simulink model "Simulation_model_full"  (R2021a)
settings: Solver=ode23t  StartTime=0.0  StopTime=6  FixedStep=T  RelTol=1e-3
values from neighbouring files (symbols this model uses):
  C_dc = Cb*c_dc_pu    [parameters.m]
  C_f = Cb*c_f_pu    [parameters.m]
  f_SM = fb    (= 50)    [parameters.m]
  fb = 50    [parameters.m]
  ff_SM = 0.01322    [parameters.m]
  Ib = 2/3*Sb/Vb    [parameters.m]
  Ib_dc = Sb/Vb_dc    [parameters.m]
  ic_SM = 0.8    [parameters.m]
  K_ad = 1.5    [parameters.m]
  K_ffv = 0    [parameters.m]
  K_ic = K_pc/T_1    [parameters.m]
  K_idc = K_pdc/T_idc    (= 250)    [parameters.m]
  K_iPLL = a^2*T_fPLL    (= 0.09)    [parameters.m]
  K_iv = K_pv/T_iv    (= 92.0050761421)    [parameters.m]
  K_iv_SM = K_pv_SM/T_iv_SM    (= 70)    [parameters.m]
  K_omega = 20    [parameters.m]
  K_omega_SM = 40    [parameters.m]
  K_pc = l_f_pu/(4*pi*fb*T_sum)    (= 1.27323954474)    [parameters.m]
  K_pdc = 25    [parameters.m]
  K_pPLL = 1/(a*2*pi*T_fPLL)    (= 5.30516476973)    [parameters.m]
  K_pv = 0.29    [parameters.m]
  K_pv_SM = 35    [parameters.m]
  K_vco = 2*pi    (= 6.28318530718)    [parameters.m]
  Kd = 40    [parameters.m]
  Kq = 0.1    [parameters.m]
  Kq_SM = 0.1    [parameters.m]
  L_f = Lb*l_f_pu    [parameters.m]
  l_f_pu = 0.08    [parameters.m]
  lfd_SM = 0.531    [parameters.m]
  llkd = 2.655    [parameters.m]
  llkq1 = 0.2408    [parameters.m]
  lls_SM = 0.08    [parameters.m]
  lmd_SM = 2.81    [parameters.m]
  lmq_SM = 1.64    [parameters.m]
  omega_ad = 50    [parameters.m]
  omega_b = 2*pi*fb    (= 314.159265359)    [parameters.m]
  omega_d = 5    [parameters.m]
  omega_qf = 200    [parameters.m]
  omega_qf_SM = 200    [parameters.m]
  omega_vf = 200    [parameters.m]
  p_h = 0.1    [parameters.m]
  pp_SM = 2    [parameters.m]
  R_lf = Rb*r_lf_pu    [parameters.m]
  rfd_SM = 0.004319    [parameters.m]
  rkd = 0.2343    [parameters.m]
  rkq1 = 0.03365    [parameters.m]
  rs_SM = 0.01524    [parameters.m]
  S_SM = Sb    (= 1000000)    [parameters.m]
  Sb = 1e6    (= 1000000)    [parameters.m]
  T = 1e-4    (= 0.0001)    [parameters.m]
  T_fPLL = 10e-3    (= 0.01)    [parameters.m]
  T_gt_SM = 0.5    [parameters.m]
  Ta = 4    [parameters.m]
  V_dc_bat = 1200    [parameters.m]
  v_dc_ref = 1    [parameters.m]
  V_SM = V    (= 690)    [parameters.m]
  Vb = V*sqrt(2)/sqrt(3)    [parameters.m]
  Vb_dc = Vb*2    [parameters.m]
undefined symbols (not defined in the file or in its folder): D1, Delta
libraries: simulink_extras x36, spsDiodeLib x24, spsThreePhaseVIMeasurementLib x16, spsThreePhaseSeriesRLCBranchLib x14, spsPower3phInstantaneousLib x8, spsVoltageMeasurementLib x5, spsControlledCurrentSourceLib x4, spsUniversalBridgeLib x4, spsParallelRLCBranchLib x2, spsSeriesRLCBranchLib x2, spsSynchronousMachinepuFundamentalLib x2, spsThreePhaseParallelRLCLoadLib x2
(part 1 of 3)
settings Model: Creator=HLunn  LastModifiedBy=HLunn

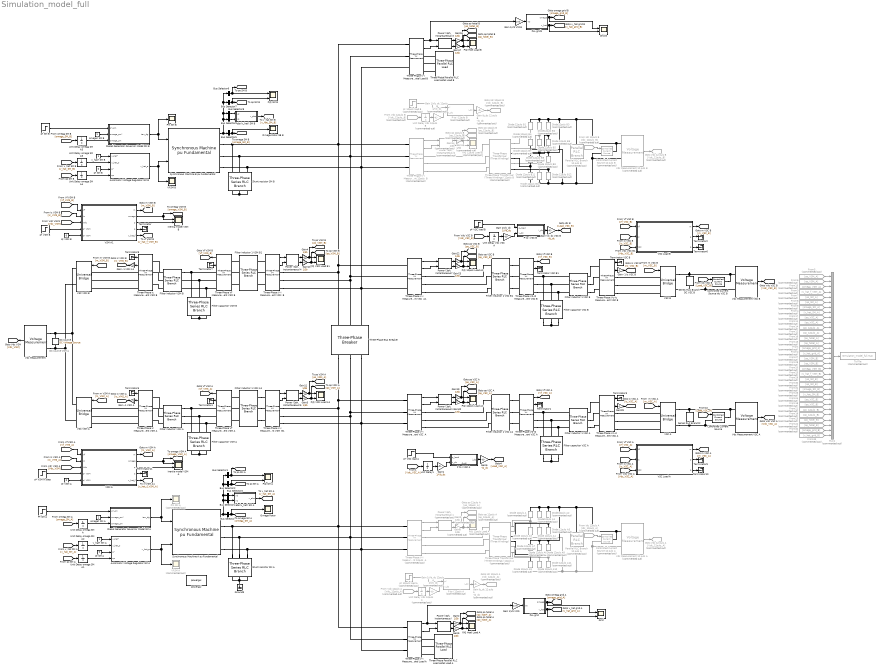
== system Simulation_model_full ==
  note: DC source
      | VSM A
  Automatic Voltage Regulator SM A : Subsystem
  Automatic Voltage Regulator SM B : Subsystem
  Bus Selector : BusSelector  OutputSignals="Mechanical.Rotor speed  wm (pu)"  OutputAsBus=on
  Bus Selector1 : BusSelector  OutputSignals="Output active power   Peo (pu)"  OutputAsBus=on
  Bus Selector2 : BusSelector  OutputSignals="Output reactive power  Qeo (pu)"  OutputAsBus=on
  Bus Selector3 : BusSelector  OutputSignals="dq0 components.Stator voltage  vd (pu)"  OutputAsBus=on
  Bus Selector4 : BusSelector  OutputSignals="dq0 components.Stator voltage  vq (pu)"  OutputAsBus=on
  Bus Selector5 : BusSelector  OutputSignals="Mechanical.Rotor speed  wm (pu)"  OutputAsBus=on
  Bus Selector6 : BusSelector  OutputSignals="Output active power   Peo (pu)"  OutputAsBus=on
  Bus Selector7 : BusSelector  OutputSignals="Output reactive power  Qeo (pu)"  OutputAsBus=on
  Bus Selector8 : BusSelector  OutputSignals="dq0 components.Stator voltage  vd (pu)"  OutputAsBus=on
  Bus Selector9 : BusSelector  OutputSignals="dq0 components.Stator voltage  vq (pu)"  OutputAsBus=on
  Controlled Current Source : spsControlledCurrentSourceLib/Controlled Current Source  Initialize=on  Source_Type=DC  Amplitude=0  Phase=0  Frequency=0  Measurements=None
  Controlled Current Source 12 puls A : spsControlledCurrentSourceLib/Controlled Current Source  Commented=on  Initialize=on  Source_Type=DC  Amplitude=0  Phase=0  Frequency=0  Measurements=None
  Controlled Current Source 12 puls B : spsControlledCurrentSourceLib/Controlled Current Source  Commented=on  Initialize=on  Source_Type=DC  Amplitude=0  Phase=0  Frequency=0  Measurements=None
  Controlled Current Source Idc VSC B : spsControlledCurrentSourceLib/Controlled Current Source  Initialize=on  Source_Type=DC  Amplitude=0  Phase=0  Frequency=0  Measurements=None
  DC source : spsDCVoltageSourceLib/DC Voltage Source  Amplitude=V_dc_bat  Measurements=None
  Diesel Generator Governor Model SM A : Subsystem
  Diesel Generator Governor Model SM B : Subsystem
  Diode 12puls A{,3..11} (10 alike) : spsDiodeLib/Diode  Commented=on  Ron=0.001  Lon=0  Vf=0.8  IC=0  UseSnubber=0  Rs=500  Cs=250e-9  Measurements=off
  Diode 12puls B{1,4..12} (10 alike) : spsDiodeLib/Diode  Commented=on  Ron=0.001  Lon=0  Vf=0.8  IC=0  UseSnubber=0  Rs=500  Cs=250e-9  Measurements=off
  Diode12puls A1 : spsDiodeLib/Diode  Commented=on  Ron=0.001  Lon=0  Vf=0.8  IC=0  UseSnubber=0  Rs=500  Cs=250e-9  Measurements=off
  Diode12puls A2 : spsDiodeLib/Diode  Commented=on  Ron=0.001  Lon=0  Vf=0.8  IC=0  UseSnubber=0  Rs=500  Cs=250e-9  Measurements=off
  Diode12puls B2 : spsDiodeLib/Diode  Commented=on  Ron=0.001  Lon=0  Vf=0.8  IC=0  UseSnubber=0  Rs=500  Cs=250e-9  Measurements=off
  Diode12puls B3 : spsDiodeLib/Diode  Commented=on  Ron=0.001  Lon=0  Vf=0.8  IC=0  UseSnubber=0  Rs=500  Cs=250e-9  Measurements=off
  Filter capacitor VSC A : spsThreePhaseSeriesRLCBranchLib/Three-Phase Series RLC Branch  LConnTagsString=A|B|C  RConnTagsString=A|B|C  BranchType=C  Resistance=R_lf*0  Inductance=L_f  Capacitance=C_f  Measurements=None
  Filter capacitor VSC B : spsThreePhaseSeriesRLCBranchLib/Three-Phase Series RLC Branch  LConnTagsString=A|B|C  RConnTagsString=A|B|C  BranchType=C  Resistance=R_lf*0  Inductance=L_f  Capacitance=C_f  Measurements=None
  Filter capacitor VSM A : spsThreePhaseSeriesRLCBranchLib/Three-Phase Series RLC Branch  LConnTagsString=A|B|C  RConnTagsString=A|B|C  BranchType=C  Resistance=R_lf*0  Inductance=L_f  Capacitance=C_f  Measurements=None
  Filter capacitor VSM B : spsThreePhaseSeriesRLCBranchLib/Three-Phase Series RLC Branch  LConnTagsString=A|B|C  RConnTagsString=A|B|C  BranchType=C  Resistance=R_lf*0  Inductance=L_f  Capacitance=C_f  Measurements=None
  Filter inductor VSM A : spsThreePhaseSeriesRLCBranchLib/Three-Phase Series RLC Branch  LConnTagsString=A|B|C  RConnTagsString=A|B|C  BranchType=RL  Resistance=R_lf  Inductance=L_f  Capacitance=1e-6  Measurements=None
  Filter inductor VSM B : spsThreePhaseSeriesRLCBranchLib/Three-Phase Series RLC Branch  LConnTagsString=A|B|C  RConnTagsString=A|B|C  BranchType=RL  Resistance=R_lf  Inductance=L_f  Capacitance=1e-6  Measurements=None
  Filter inductor 1 VSC A : spsThreePhaseSeriesRLCBranchLib/Three-Phase Series RLC Branch  LConnTagsString=A|B|C  RConnTagsString=A|B|C  BranchType=RL  Resistance=R_lf  Inductance=L_f  Capacitance=1e-6  Measurements=None
  Filter inductor 1 VSC A1 : spsThreePhaseSeriesRLCBranchLib/Three-Phase Series RLC Branch  LConnTagsString=A|B|C  RConnTagsString=A|B|C  BranchType=RL  Resistance=R_lf  Inductance=L_f  Capacitance=1e-6  Measurements=None
  Filter inductor 1 VSC B : spsThreePhaseSeriesRLCBranchLib/Three-Phase Series RLC Branch  LConnTagsString=A|B|C  RConnTagsString=A|B|C  BranchType=RL  Resistance=R_lf  Inductance=L_f  Capacitance=1e-6  Measurements=None
  Filter inductor 1 VSC B1 : spsThreePhaseSeriesRLCBranchLib/Three-Phase Series RLC Branch  LConnTagsString=A|B|C  RConnTagsString=A|B|C  BranchType=RL  Resistance=R_lf  Inductance=L_f  Capacitance=1e-6  Measurements=None
  Filter inductor 1 VSM A1 : spsThreePhaseSeriesRLCBranchLib/Three-Phase Series RLC Branch  LConnTagsString=A|B|C  RConnTagsString=A|B|C  BranchType=RL  Resistance=R_lf  Inductance=L_f  Capacitance=1e-6  Measurements=None
  Filter inductor 1 VSM B1 : spsThreePhaseSeriesRLCBranchLib/Three-Phase Series RLC Branch  LConnTagsString=A|B|C  RConnTagsString=A|B|C  BranchType=RL  Resistance=R_lf  Inductance=L_f  Capacitance=1e-6  Measurements=None
  From : From  Commented=on  GotoTag=omega_grid_A
  From Idc 12puls A : From  Commented=on  GotoTag=Idc_12puls_A
  From Idc 12puls B : From  Commented=on  GotoTag=Idc_12puls_B
  From Vdc 12puls A : From  Commented=on  GotoTag=Vdc_12puls_A
  From Vdc 12puls B : From  Commented=on  GotoTag=Vdc_12puls_B
  From11 : From  Commented=on  GotoTag=qo_VSC_A
  From12 : From  Commented=on  GotoTag=qo_12puls_A
  From13 : From  Commented=on  GotoTag=omega_VSM_A
  From14 : From  Commented=on  GotoTag=po_12puls_A
  From15 : From  Commented=on  GotoTag=qo_hotel_A
  From16 : From  Commented=on  GotoTag=po_hotel_A
  From17 : From  Commented=on  GotoTag=po_VSC_A
  From18 : From  Commented=on  GotoTag=qo_VSC_B
  From19 : From  Commented=on  GotoTag=qo_12puls_B
  From2 : From  Commented=on  GotoTag=v_hat_grid_A
  From20 : From  Commented=on  GotoTag=omega_VSM_B
  From21 : From  Commented=on  GotoTag=po_12puls_B
  From22 : From  Commented=on  GotoTag=qo_hotel_B
  From23 : From  Commented=on  GotoTag=po_hotel_B
  From24 : From  Commented=on  GotoTag=po_VSC_B
  From25 : From  Commented=on  GotoTag=v_hat_f_VSM_B
  From26 : From  Commented=on  GotoTag=v_hat_SM_B
  From27 : From  Commented=on  GotoTag=po_VSM_B
  From28 : From  Commented=on  GotoTag=qo_VSM_B
  From29 : From  Commented=on  GotoTag=po_SM_B
  From3 : From  Commented=on  GotoTag=v_hat_f_VSM_A
  From30 : From  Commented=on  GotoTag=qo_SM_B
  From31 : From  Commented=on  GotoTag=omega_SM_B
  From32 : From  Commented=on  GotoTag=omega_grid_B
  From33 : From  Commented=on  GotoTag=v_hat_grid_B
  From4 : From  Commented=on  GotoTag=v_hat_SM_A
  From5 : From  Commented=on  GotoTag=po_VSM_A
  From6 : From  Commented=on  GotoTag=qo_VSM_A
  From7 : From  Commented=on  GotoTag=po_SM_A
  From8 : From  Commented=on  GotoTag=qo_SM_A
  From9 : From  Commented=on  GotoTag=omega_SM_A
  Gain -1 Ic VSC B : Gain  Gain=-1
  Gain -1 VSM A : Gain  Gain=-1
  Gain -1 VSM A1 : Gain  Gain=-1
  Gain 1/Vb VMS : Gain  Gain=1/Vb
  Gain 1/Vb VMS1 : Gain  Gain=1/Vb
  Gain 1/Vb_dc : Gain  Gain=1/Vb_dc
  Gain 1/Vb_dc 12puls A : Gain  Commented=on  Gain=1/Vb_dc
  Gain 1/Vb_dc 12puls B : Gain  Commented=on  Gain=1/Vb_dc
  Gain Ib_dc 12 puls A : Gain  Commented=on  Gain=-Ib_dc
  Gain Ib_dc 12 puls B : Gain  Commented=on  Gain=-Ib_dc
  Gain Vb_dc VSC B : Gain  Gain=-Ib_dc
  Gain1 : Gain  Gain=1/Vb_dc
  Gain{2..5,10..11,16..17,19..20,22..23} (12 alike) : Gain  Gain=1/Sb
  Gain{8..9,13..14} (4 alike) : Gain  Commented=on  Gain=1/Sb
  Gain29 : Gain  Gain=-1
  Gain6 : Gain  Gain=-Ib_dc
  Goto Idc 12puls A : Goto  Commented=on  GotoTag=Idc_12puls_A
  Goto Idc 12puls B : Goto  Commented=on  GotoTag=Idc_12puls_B
  Goto Vdc 12 puls A : Goto  Commented=on  GotoTag=Vdc_12puls_A
  Goto Vdc 12 puls B : Goto  Commented=on  GotoTag=Vdc_12puls_B
  Goto po 12puls A : Goto  Commented=on  GotoTag=po_12puls_A
  Goto po 12puls B : Goto  Commented=on  GotoTag=po_12puls_B
  Goto qo 12puls A : Goto  Commented=on  GotoTag=qo_12puls_A
  Goto qo 12puls B : Goto  Commented=on  GotoTag=qo_12puls_B
  Grid : Scope  NumInputPorts=2
  Grid B : Scope  NumInputPorts=2
  Ground3 : spsGroundLib/Ground  LConnTagsString=a
  Inertia model VSM A : Scope  NumInputPorts=2
  Inertia model VSM B : Scope  NumInputPorts=2
  Mux1 : Mux  Commented=on  Inputs=32
  Omega Rotor : Scope
  Omega Rotor SB B : Scope
  P to I VSC A : Subsystem
      settings: PortSchema="{\"entries\":[{\"content\":{\"sides\":[{\"content\":{\"connectorIds\":[\"In1\",\"In2\"]},\"type\":\"ConnectorPlacement.EquallySpacedRectSide\",\"uuid\":\"1b3d670f-a973-44e5-93e0-282aed06b720\"},{\"content\":{\"connectorIds\":[\"Out1\"],\"side\":\"RIGHT\"},\"type\":\"ConnectorPlacement.EquallySpacedRectSide\",\"uuid\":\"c6dbaf48-01df-4046-a8d4-fcaf539dec06\"},{\"content\":{\"connectorIds\":[],\"side\":\"TOP\"},\"type\":\"ConnectorPlacement.EquallySpacedRectSide\",\"uuid\":\"017adae8-c967-4395-bb40-0db2b451d960\"},{\"content\":{\"connectorIds\":[\"Out2\"],\"side\":\"BOTTOM\"},\"type\":\"ConnectorPlacement.EquallySpacedRectSide\",\"uuid\":\"114f5234-785a-4230-ad61-b1c2a38e27d5\"}]},\"type\":\"ConnectorPlacement.EquallySpacedConnector\",\"uuid\":\"a79c07b6-0122-49d2-8cca-a205e7e92776\"}],\"packageUris\":[\"http://schema.mathworks.com/mf0/Connector/R2020b\"],\"version\":\"1.0\"}"
  P to I VSC B : Subsystem
  P to I 12puls A : Subsystem  Commented=on
  P to I 12puls B : Subsystem  Commented=on
  "P* SM A " : Step  Time=2  Before=0.05  After=0.2  SampleTime=0
  P/Q 12puls Load A : Scope  Commented=on  NumInputPorts=2
  P/Q 12puls Load A1 : Scope  NumInputPorts=2
  P/Q 12puls Load A2 : Scope  NumInputPorts=2
  P/Q 12puls Load B : Scope  Commented=on  NumInputPorts=2
  P/Q Hoel Load A : Scope  NumInputPorts=2
  P/Q Hoel Load B : Scope  NumInputPorts=2
  P/Q SM A : Scope  NumInputPorts=2
  P/Q SM B : Scope  NumInputPorts=2
  P/Q VSM Load A1 : Scope  NumInputPorts=2
  P/Q VSM Load B1 : Scope  NumInputPorts=2
  PLL grid : Subsystem
  PLL grid1 : Subsystem
  Parallel RLC Branch 12 puls A : spsParallelRLCBranchLib/Parallel RLC Branch  Commented=on  LConnTagsString=a  RConnTagsString=__new0  BranchType=C  Resistance=1e3  Inductance=1e-3  SetiL0=off  InitialCurrent=0  Capacitance=C_dc  Setx0=on  InitialVoltage=Vb_dc  Measurements=None
  Parallel RLC Branch 12 puls B : spsParallelRLCBranchLib/Parallel RLC Branch  Commented=on  LConnTagsString=a  RConnTagsString=__new0  BranchType=C  Resistance=1e3  Inductance=1e-3  SetiL0=off  InitialCurrent=0  Capacitance=C_dc  Setx0=on  InitialVoltage=Vb_dc  Measurements=None
  Pm SM A : Scope  Commented=on
  Pm SM B : Scope
  Power (3ph, Instantaneous){,3..7} (6 alike) : spsPower3phInstantaneousLib/Power (3ph, Instantaneous)
  "Power (3ph, Instantaneous)1" : spsPower3phInstantaneousLib/Power (3ph, Instantaneous)  Commented=on
  "Power (3ph, Instantaneous)2" : spsPower3phInstantaneousLib/Power (3ph, Instantaneous)  Commented=on
  Series RLC Branch DC VSC B : spsSeriesRLCBranchLib/Series RLC Branch  LConnTagsString=__new0  RConnTagsString=__new0  BranchType=C  Resistance=0  Inductance=0  SetiL0=off  InitialCurrent=0  Capacitance=C_dc  Setx0=on  InitialVoltage=Vb_dc  Measurements=None
  Series RLC Branch2 : spsSeriesRLCBranchLib/Series RLC Branch  LConnTagsString=__new0  RConnTagsString=__new0  BranchType=C  Resistance=0  Inductance=0  SetiL0=off  InitialCurrent=0  Capacitance=C_dc  Setx0=on  InitialVoltage=Vb_dc  Measurements=None
  Shunt resistor SM A : spsThreePhaseSeriesRLCBranchLib/Three-Phase Series RLC Branch  LConnTagsString=A|B|C  RConnTagsString=A|B|C  BranchType=R  Resistance=1e6  Inductance=L_f  Capacitance=C_f  Measurements=None
  Shunt resistor SM B : spsThreePhaseSeriesRLCBranchLib/Three-Phase Series RLC Branch  LConnTagsString=A|B|C  RConnTagsString=A|B|C  BranchType=R  Resistance=1e6  Inductance=L_f  Capacitance=C_f  Measurements=None
  Synchronous Machine A pu Fundamental : spsSynchronousMachinepuFundamentalLib/Synchronous Machine pu Fundamental  PresetModel=No  MechanicalLoad=Mechanical power Pm  ShowDetailedParameters=on  RotorType=Salient-pole  Units=per unit fundamental parameters  MeasurementBus=off  NominalParameters=[S_SM V_SM f_SM]  Stator=[rs_SM lls_SM lmd_SM lmq_SM]  Field=[rfd_SM lfd_SM]  Dampers2=[0.0652, 0.5134, 0.0287, 0.2553, 7.765e-3, 0.9167 ]  Dampers1=[rkd llkd rkq1 llkq1]  Mechanical=[ic_SM ff_SM pp_SM]  PolePairs=20  InitialConditions="[ 0  0  0  0  0  0  0  0  1 ]"  SetSaturation=off  Saturation=[0.6404,0.7127,0.8441,0.9214,0.9956,1.082,1.19,1.316,1.457;0.7,0.7698,0.8872,0.9466,0.9969,1.046,1.1,1.151,1.201]  LoadFlowParameters=[1,0,0,0,0]  TsPowergui=0  TsBlock=-1  IterativeModel=Trapezoidal non iterative  IterativeDiscreteModel=Trapezoidal non iterative  BusType=PV  Pref=0  Qref=0  Qmin=-inf  Qmax=inf  PLF=0  QLF=0
      settings: SourceProductBaseCode=PS
  Synchronous Machine B pu Fundamental : spsSynchronousMachinepuFundamentalLib/Synchronous Machine pu Fundamental  PresetModel=No  MechanicalLoad=Mechanical power Pm  ShowDetailedParameters=on  RotorType=Salient-pole  Units=per unit fundamental parameters  MeasurementBus=off  NominalParameters=[S_SM V_SM f_SM]  Stator=[rs_SM lls_SM lmd_SM lmq_SM]  Field=[rfd_SM lfd_SM]  Dampers2=[0.0652, 0.5134, 0.0287, 0.2553, 7.765e-3, 0.9167 ]  Dampers1=[rkd llkd rkq1 llkq1]  Mechanical=[ic_SM ff_SM pp_SM]  PolePairs=20  InitialConditions="[ 0  0  0  0  0  0  0  0  1 ]"  SetSaturation=off  Saturation=[0.6404,0.7127,0.8441,0.9214,0.9956,1.082,1.19,1.316,1.457;0.7,0.7698,0.8872,0.9466,0.9969,1.046,1.1,1.151,1.201]  LoadFlowParameters=[1,0,0,0,0]  TsPowergui=0  TsBlock=-1  IterativeModel=Trapezoidal non iterative  IterativeDiscreteModel=Trapezoidal non iterative  BusType=PV  Pref=0  Qref=0  Qmin=-inf  Qmax=inf  PLF=0  QLF=0
      settings: SourceProductBaseCode=PS
  Terminator{,1..11} (12 alike) : Terminator
  Terminator VSC B : Terminator
  Terminator VSC B1 : Terminator
  Three-Phase Ic Measurement VSM A : spsThreePhaseVIMeasurementLib/Three-Phase V-I Measurement  VoltageMeasurement=phase-to-ground  SetLabelV=off  LabelV=V_cv  Vpu=off  VpuLL=off  CurrentMeasurement=yes  SetLabelI=off  LabelI=I_cv  Ipu=off  Pbase=Sb  Vbase=V  OutputType=Complex  PhasorSimulation=off  PSBequivalent=0
  Three-Phase Ic Measurement VSM B : spsThreePhaseVIMeasurementLib/Three-Phase V-I Measurement  VoltageMeasurement=phase-to-ground  SetLabelV=off  LabelV=V_cv  Vpu=off  VpuLL=off  CurrentMeasurement=yes  SetLabelI=off  LabelI=I_cv  Ipu=off  Pbase=Sb  Vbase=V  OutputType=Complex  PhasorSimulation=off  PSBequivalent=0
  Three-Phase Parallel RLC Load Hotel Load A : spsThreePhaseParallelRLCLoadLib/Three-Phase Parallel RLC Load  LConnTagsString=A|B|C  Configuration=Y (floating)  NominalVoltage=690  Vabc=[1e3 1e3 1e3]  Vabcp=[1e3 1e3 1e3]  NominalFrequency=fb  UnbalancedPower=off  ActivePower=Sb*p_h  InductivePower=0  CapacitivePower=0  Pabc=[10e3 9e3 11e3]  QLabc=[100 90 110]  QCabc=[100 90 110]  Pabcp=[10e3 9e3 11e3]  QLabcp=[100 90 110]  QCabcp=[100 90 110]  Measurements=None  LoadType=constant Z
  Three-Phase Parallel RLC Load Hotel Load B : spsThreePhaseParallelRLCLoadLib/Three-Phase Parallel RLC Load  LConnTagsString=A|B|C  Configuration=Y (floating)  NominalVoltage=690  Vabc=[1e3 1e3 1e3]  Vabcp=[1e3 1e3 1e3]  NominalFrequency=fb  UnbalancedPower=off  ActivePower=Sb*p_h  InductivePower=0  CapacitivePower=0  Pabc=[10e3 9e3 11e3]  QLabc=[100 90 110]  QCabc=[100 90 110]  Pabcp=[10e3 9e3 11e3]  QLabcp=[100 90 110]  QCabcp=[100 90 110]  Measurements=None  LoadType=constant Z
  Three-Phase Transformer (Three Windings) 12puls A : spsThreePhaseTransformerThreeWindingsLib/Three-Phase Transformer (Three Windings)  Commented=on  Winding1Connection=Y  Winding2Connection=Y  Winding3Connection=Delta (D1)  CoreType=Three single-phase transformers  SetSaturation=off  Hysteresis=off  DataFile='hysteresis'  SetInitialFlux=off  Measurements=None  UNITS=pu  NominalPower=[Sb , fb]  Winding1=[690 0.005 0.04]  Winding2=[690 0.005 0.03]  Winding3=[690 0.005 0.03]  Rm=100  Lm=100  L0=0.5  Saturation=[0 0;2.2531e-06 1278.3;0.00093879 1619.1]  InitialFluxes=[0.8 -0.8 0.7]  BreakLoop=off  DiscreteSolver=Trapezoidal iterative  DataType=off  TransfoNumber=1
      settings: SourceProductBaseCode=PS
  Three-Phase Transformer (Three Windings) 12puls B : spsThreePhaseTransformerThreeWindingsLib/Three-Phase Transformer (Three Windings)  Commented=on  Winding1Connection=Y  Winding2Connection=Y  Winding3Connection=Delta (D1)  CoreType=Three single-phase transformers  SetSaturation=off  Hysteresis=off  DataFile='hysteresis'  SetInitialFlux=off  Measurements=None  UNITS=pu  NominalPower=[Sb , fb]  Winding1=[690 0.005 0.04]  Winding2=[690 0.005 0.03]  Winding3=[690 0.005 0.03]  Rm=100  Lm=100  L0=0.5  Saturation=[0 0;2.2531e-06 1278.3;0.00093879 1619.1]  InitialFluxes=[0.8 -0.8 0.7]  BreakLoop=off  DiscreteSolver=Trapezoidal iterative  DataType=off  TransfoNumber=1
      settings: SourceProductBaseCode=PS
  Three-Phase V-I Measurement 12puls  A : spsThreePhaseVIMeasurementLib/Three-Phase V-I Measurement  Commented=on  VoltageMeasurement=phase-to-ground  SetLabelV=off  LabelV=Vabc  Vpu=off  VpuLL=off  CurrentMeasurement=yes  SetLabelI=off  LabelI=Iabc  Ipu=off  Pbase=100e6  Vbase=500e3  OutputType=Complex  PhasorSimulation=off  PSBequivalent=0
  Three-Phase V-I Measurement 12puls  B : spsThreePhaseVIMeasurementLib/Three-Phase V-I Measurement  Commented=on  VoltageMeasurement=phase-to-ground  SetLabelV=off  LabelV=Vabc  Vpu=off  VpuLL=off  CurrentMeasurement=yes  SetLabelI=off  LabelI=Iabc  Ipu=off  Pbase=100e6  Vbase=500e3  OutputType=Complex  PhasorSimulation=off  PSBequivalent=0
  Three-Phase V-I Measurement Hotel Load A : spsThreePhaseVIMeasurementLib/Three-Phase V-I Measurement  VoltageMeasurement=phase-to-ground  SetLabelV=off  LabelV=Vabc  Vpu=off  VpuLL=off  CurrentMeasurement=yes  SetLabelI=off  LabelI=Iabc  Ipu=off  Pbase=100e6  Vbase=500e3  OutputType=Complex  PhasorSimulation=off  PSBequivalent=0
  Three-Phase V-I Measurement Hotel Load B : spsThreePhaseVIMeasurementLib/Three-Phase V-I Measurement  VoltageMeasurement=phase-to-ground  SetLabelV=off  LabelV=Vabc  Vpu=off  VpuLL=off  CurrentMeasurement=yes  SetLabelI=off  LabelI=Iabc  Ipu=off  Pbase=100e6  Vbase=500e3  OutputType=Complex  PhasorSimulation=off  PSBequivalent=0
  Three-Phase V-I Measurement VSC  A : spsThreePhaseVIMeasurementLib/Three-Phase V-I Measurement  VoltageMeasurement=phase-to-ground  SetLabelV=off  LabelV=Vabc  Vpu=off  VpuLL=off  CurrentMeasurement=yes  SetLabelI=off  LabelI=Iabc  Ipu=off  Pbase=100e6  Vbase=500e3  OutputType=Complex  PhasorSimulation=off  PSBequivalent=0
  Three-Phase V-I Measurement VSC  A1 : spsThreePhaseVIMeasurementLib/Three-Phase V-I Measurement  VoltageMeasurement=phase-to-ground  SetLabelV=off  LabelV=Vabc  Vpu=off  VpuLL=off  CurrentMeasurement=yes  SetLabelI=off  LabelI=Iabc  Ipu=off  Pbase=100e6  Vbase=500e3  OutputType=Complex  PhasorSimulation=off  PSBequivalent=0
  Three-Phase V-I Measurement VSM  B : spsThreePhaseVIMeasurementLib/Three-Phase V-I Measurement  VoltageMeasurement=phase-to-ground  SetLabelV=off  LabelV=Vabc  Vpu=off  VpuLL=off  CurrentMeasurement=yes  SetLabelI=off  LabelI=Iabc  Ipu=off  Pbase=100e6  Vbase=500e3  OutputType=Complex  PhasorSimulation=off  PSBequivalent=0
  Three-Phase V-I Measurement VSM  B1 : spsThreePhaseVIMeasurementLib/Three-Phase V-I Measurement  VoltageMeasurement=phase-to-ground  SetLabelV=off  LabelV=Vabc  Vpu=off  VpuLL=off  CurrentMeasurement=yes  SetLabelI=off  LabelI=Iabc  Ipu=off  Pbase=100e6  Vbase=500e3  OutputType=Complex  PhasorSimulation=off  PSBequivalent=0
  Three-Phase V0-I0 Measurement VSC A : spsThreePhaseVIMeasurementLib/Three-Phase V-I Measurement  VoltageMeasurement=phase-to-ground  SetLabelV=off  LabelV=Vabc  Vpu=off  VpuLL=off  CurrentMeasurement=yes  SetLabelI=off  LabelI=Iabc  Ipu=off  Pbase=100e6  Vbase=500e3  OutputType=Complex  PhasorSimulation=off  PSBequivalent=0
  Three-Phase V0-I0 Measurement VSC B : spsThreePhaseVIMeasurementLib/Three-Phase V-I Measurement  VoltageMeasurement=phase-to-ground  SetLabelV=off  LabelV=Vabc  Vpu=off  VpuLL=off  CurrentMeasurement=yes  SetLabelI=off  LabelI=Iabc  Ipu=off  Pbase=100e6  Vbase=500e3  OutputType=Complex  PhasorSimulation=off  PSBequivalent=0
  Three-Phase Vc-Ic Measurement VSC A : spsThreePhaseVIMeasurementLib/Three-Phase V-I Measurement  VoltageMeasurement=phase-to-ground  SetLabelV=off  LabelV=V_cv  Vpu=off  VpuLL=off  CurrentMeasurement=yes  SetLabelI=off  LabelI=I_cv  Ipu=off  Pbase=Sb  Vbase=V  OutputType=Complex  PhasorSimulation=off  PSBequivalent=0
  Three-Phase Vc-Ic Measurement VSC B : spsThreePhaseVIMeasurementLib/Three-Phase V-I Measurement  VoltageMeasurement=phase-to-ground  SetLabelV=off  LabelV=V_cv  Vpu=off  VpuLL=off  CurrentMeasurement=yes  SetLabelI=off  LabelI=I_cv  Ipu=off  Pbase=Sb  Vbase=V  OutputType=Complex  PhasorSimulation=off  PSBequivalent=0
  Three-Phase Vf Measurement VSM A : spsThreePhaseVIMeasurementLib/Three-Phase V-I Measurement  VoltageMeasurement=phase-to-ground  SetLabelV=off  LabelV=Vabc  Vpu=off  VpuLL=off  CurrentMeasurement=yes  SetLabelI=off  LabelI=Iabc  Ipu=off  Pbase=100e6  Vbase=500e3  OutputType=Complex  PhasorSimulation=off  PSBequivalent=0
  Three-Phase Vf Measurement VSM B : spsThreePhaseVIMeasurementLib/Three-Phase V-I Measurement  VoltageMeasurement=phase-to-ground  SetLabelV=off  LabelV=Vabc  Vpu=off  VpuLL=off  CurrentMeasurement=yes  SetLabelI=off  LabelI=Iabc  Ipu=off  Pbase=100e6  Vbase=500e3  OutputType=Complex  PhasorSimulation=off  PSBequivalent=0
  Three-Phase Bus Breaker : spsThreePhaseBreakerLib/Three-Phase Breaker  InitialState=closed  SwitchA=on  SwitchB=on  SwitchC=on  SwitchTimes=[100]  External=off  BreakerResistance=0.01  SnubberResistance=1e6  SnubberCapacitance=inf  Measurements=None
  To File : ToFile  Commented=on  Filename=Simulation_model_full.mat  MatrixName=Simulation_model_full
  Unit Delay Vdc 12puls A : UnitDelay  Commented=on  InitialCondition=Vb_dc  SampleTime=-1  HasFrameUpgradeWarning=on
  Unit Delay Vdc 12puls B : UnitDelay  Commented=on  InitialCondition=Vb_dc  SampleTime=-1  HasFrameUpgradeWarning=on
  Unit Delay Vdc VSC A : UnitDelay  InitialCondition=Vb_dc  SampleTime=-1  HasFrameUpgradeWarning=on
  Unit Delay omega SM A{,1..5} (6 alike) : UnitDelay  SampleTime=-1  HasFrameUpgradeWarning=on
  Unit Delay1 : UnitDelay  InitialCondition=Vb_dc  SampleTime=-1  HasFrameUpgradeWarning=on
  VSC A : spsUniversalBridgeLib/Universal Bridge  Arms=3  SnubberResistance=1e5  SnubberCapacitance=inf  Device=Average-model based VSC  Ron=1e-3  Lon=0  ForwardVoltages="[  0  0  ]"  ForwardVoltage=0  GTOparameters=[ 10e-6 , 20e-6 ]  IGBTparameters=[ 1e-6 , 2e-6 ]  Measurements=None  Measurements_2=None  converterType=Rectifier
  VSC B : spsUniversalBridgeLib/Universal Bridge  Arms=3  SnubberResistance=1e5  SnubberCapacitance=inf  Device=Average-model based VSC  Ron=1e-3  Lon=0  ForwardVoltages="[  0  0  ]"  ForwardVoltage=0  GTOparameters=[ 10e-6 , 20e-6 ]  IGBTparameters=[ 1e-6 , 2e-6 ]  Measurements=None  Measurements_2=None  converterType=Rectifier
  VSC Load A : Subsystem
  VSC Load B : Subsystem
  VSC VSM A : spsUniversalBridgeLib/Universal Bridge  Arms=3  SnubberResistance=1e5  SnubberCapacitance=inf  Device=Average-model based VSC  Ron=1e-3  Lon=0  ForwardVoltages="[  0  0  ]"  ForwardVoltage=0  GTOparameters=[ 10e-6 , 20e-6 ]  IGBTparameters=[ 1e-6 , 2e-6 ]  Measurements=None  Measurements_2=None  converterType=Rectifier
  VSC VSM B : spsUniversalBridgeLib/Universal Bridge  Arms=3  SnubberResistance=1e5  SnubberCapacitance=inf  Device=Average-model based VSC  Ron=1e-3  Lon=0  ForwardVoltages="[  0  0  ]"  ForwardVoltage=0  GTOparameters=[ 10e-6 , 20e-6 ]  IGBTparameters=[ 1e-6 , 2e-6 ]  Measurements=None  Measurements_2=None  converterType=Rectifier
  VSM A : Subsystem
  VSM A1 : Subsystem
  Vdc Measurement : spsVoltageMeasurementLib/Voltage Measurement  PhasorSimulation=off  OutputType=Complex  PSBequivalent=0
  Vdc Measurement 12 puls A : spsVoltageMeasurementLib/Voltage Measurement  Commented=on  PhasorSimulation=off  OutputType=Complex  PSBequivalent=0
  Vdc Measurement 12 puls B : spsVoltageMeasurementLib/Voltage Measurement  Commented=on  PhasorSimulation=off  OutputType=Complex  PSBequivalent=0
  Vdc Measurement VSC A : spsVoltageMeasurementLib/Voltage Measurement  PhasorSimulation=off  OutputType=Complex  PSBequivalent=0
  Vdc Measurement VSC B : spsVoltageMeasurementLib/Voltage Measurement  PhasorSimulation=off  OutputType=Complex  PSBequivalent=0
  Vf SM A : Scope  Commented=on
  Vf SM B : Scope
  abs(v_hat) SM A : MATLAB Function  TreatAsAtomicUnit=on
  abs(v_hat) SM B : MATLAB Function  TreatAsAtomicUnit=on
  omega* SM A : Constant
  omega* SM B : Constant
  p* 12puls load A : Step  Commented=on  Time=2  After=0.3  SampleTime=0
  "p* 12puls load B   " : Step  Commented=on  Time=2  After=0.3  SampleTime=0
  p* SM B : Step  Time=2  Before=0.05  After=0.2  SampleTime=0
  p* VSC load A : Step  Time=2  After=0.3  SampleTime=0
  "p* VSC load B " : Step  Time=2  After=0.3  SampleTime=0
  p* VSM A step : Step  Time=2  Before=0.05  After=0.2  SampleTime=0
  "p* VSM B " : Step  Time=2  Before=0.05  After=0.2  SampleTime=0
  powergui : spspowerguiLib/powergui  Priority=1  SimulationMode=Discrete  SampleTime=T  frequency=60  Iterations=50  frequencyindice=50  Pbase=100e6  ErrMax=1e-4  UnitsV=kV  UnitsW=MW  buscounter=0  FunctionMessages=off  echomessages=off  EnableUseOfTLC=off  CurrentSourceSwitches=off  DisableSnubberDevices=off  DisableRonSwitches=off  DisableVfSwitches=off  DisplayEquations=off  AutomaticDiscreteSolvers=off  SolverType=Tustin/Backward Euler (TBE)  Interpol=off  ExternalGateDelay=off  methode=off  Ts=100  x0status=blocks  SPID=on  SwTol=0  HookPort=off  NonlinearTolerance=1e-4  nMaxIteration=100  ContinueOnMaxIteration=off  RestoreLinks=warning  ResistiveCurrentMeasurement=off  Frange=[0:2:500]  Ylog=off  Xlog=on  ShowGrid=off  save=off  variable=ZData  structure=0  ZoomFFT=off  StartTime=0.0  cycles=1  DisplayStyle=1  fundamental=60  FreqAxis=off  MaxFrequency=1000  frequencyindicesteady=1  RmsSteady=1  display=off
  q* SM A : Constant  Value=0
  q* SM B : Constant  Value=0
  q* VSM A : Constant  Value=0
  q* VSM B : Constant  Value=0
  v_hat* SM A : Constant
  v_hat* SM B : Constant
  wires:
  [qo_SM_A] -> Unit Delay omega SM A1/1
  q* SM A/1 -> Automatic Voltage Regulator SM A/3(q*)
  v_hat* SM A/1 -> Automatic Voltage Regulator SM A/1(v_hat*)
  [v_hat_SM_A] -> Unit Delay omega SM A2/1
  omega* SM A/1 -> Diesel Generator Governor Model SM A/2(omega_sm*)
  Synchronous Machine A pu Fundamental/1 -> Bus Selector/1, Bus Selector1/1, Bus Selector2/1, Bus Selector3/1, Bus Selector4/1
  Bus Selector/1 -> Omega Rotor/1, [omega_SM_A]
  Unit Delay omega SM A/1 -> Diesel Generator Governor Model SM A/3(omega_sm)
  [omega_SM_A] -> Unit Delay omega SM A/1
  Bus Selector1/1 -> [po_SM_A], P/Q SM A/1
  Bus Selector3/1 -> abs(v_hat) SM A/1(vd)
  Bus Selector4/1 -> abs(v_hat) SM A/2(vq)
  Bus Selector2/1 -> P/Q SM A/2, [qo_SM_A]
  abs(v_hat) SM A/1(v_abs) -> [v_hat_SM_A]
  P to I 12puls A/1(i_dc) -> Gain Ib_dc 12 puls A/1
  From Idc 12puls A/1 -> Controlled Current Source 12 puls A/1
  Gain Ib_dc 12 puls A/1 -> Goto Idc 12puls A/1
  Unit Delay Vdc 12puls A/1 -> Gain 1/Vb_dc 12puls A/1
  From Vdc 12puls A/1 -> Unit Delay Vdc 12puls A/1
  p* 12puls load A/1 -> P to I 12puls A/1(p*)
  Gain 1/Vb_dc 12puls A/1 -> P to I 12puls A/2(v_dc)
  Vdc Measurement 12 puls A/1 -> Goto Vdc 12 puls A/1
  Gain6/1 -> [Load_VSC_A]
  Gain1/1 -> P to I VSC A/2(v_dc)
  P to I VSC A/1(i_dc) -> Gain6/1
  Vdc Measurement VSC A/1 -> [Vdc_VSC_A]
  Gain29/1 -> [Ic_VSC_A]
  Three-Phase V0-I0 Measurement VSC A/2 -> Terminator1/1
  Three-Phase V0-I0 Measurement VSC A/1 -> [Vf_VSC_A]
  Three-Phase Vc-Ic Measurement VSC A/1 -> Terminator3/1
  Three-Phase Vc-Ic Measurement VSC A/2 -> Gain29/1
  [Load_VSC_A] -> Controlled Current Source/1
  [m_VSC_A] -> VSC A/1
  p* VSC load A/1 -> P to I VSC A/1(p_load)
  Three-Phase Vf Measurement VSM A/1 -> [Vf_VMS_A]
  Three-Phase Ic Measurement VSM A/2 -> Gain -1 VSM A/1
  Three-Phase Vf Measurement VSM A/2 -> Terminator4/1
  Gain -1 VSM A/1 -> [Ic_VMS_A]
  Three-Phase Ic Measurement VSM A/1 -> Terminator5/1
  Vdc Measurement/1 -> [Vdc_VSM]
  [m_VSM_A] -> VSC VSM A/1
  Unit Delay omega SM A1/1 -> Automatic Voltage Regulator SM A/4(qo)
  Unit Delay omega SM A2/1 -> Automatic Voltage Regulator SM A/2(v_hat_o)
  Unit Delay1/1 -> Gain1/1
  [Vdc_VSC_A] -> Unit Delay1/1
  [Vf_VSC_A] -> VSC Load A/1(Vf)
  [Vdc_VSC_A] -> VSC Load A/3(Vdc)
  VSC Load A/1(m) -> [m_VSC_A]
  [Ic_VSC_A] -> VSC Load A/2(Ic)
  Unit Delay omega SM A4/1 -> Automatic Voltage Regulator SM B/4(qo)
  [m_VSM_B] -> VSC VSM B/1
  Three-Phase Ic Measurement VSM B/1 -> Terminator8/1
  Three-Phase Vf Measurement VSM B/2 -> Terminator7/1
  Gain -1 VSM A1/1 -> [Ic_VMS_B]
  Three-Phase Ic Measurement VSM B/2 -> Gain -1 VSM A1/1
  Three-Phase Vf Measurement VSM B/1 -> [Vf_VMS_B]
  Unit Delay omega SM A5/1 -> Automatic Voltage Regulator SM B/2(v_hat_o)
  "p* 12puls load B   "/1 -> P to I 12puls B/1(p*)
  [Vdc_VSC_B] -> Unit Delay Vdc VSC A/1
  abs(v_hat) SM B/1(v_abs) -> [v_hat_SM_B]
  "p* VSC load B "/1 -> P to I VSC B/1(p_load)
  [Ic_VSC_B] -> VSC Load B/2(Ic)
  VSC Load B/1(m) -> [m_VSC_B]
  [Vf_VSC_B] -> VSC Load B/1(Vf)
  [omega_SM_B] -> Unit Delay omega SM A3/1
  Bus Selector9/1 -> abs(v_hat) SM B/2(vq)
  Bus Selector6/1 -> [po_SM_B], P/Q SM B/1
  Unit Delay omega SM A3/1 -> Diesel Generator Governor Model SM B/3(omega_sm)
  Bus Selector5/1 -> Omega Rotor SB B/1, [omega_SM_B]
  Synchronous Machine B pu Fundamental/1 -> Bus Selector5/1, Bus Selector6/1, Bus Selector7/1, Bus Selector8/1, Bus Selector9/1
  omega* SM B/1 -> Diesel Generator Governor Model SM B/2(omega_sm*)
  Gain 1/Vb_dc/1 -> P to I VSC B/2(v_dc)
  v_hat* SM B/1 -> Automatic Voltage Regulator SM B/1(v_hat*)
  q* SM B/1 -> Automatic Voltage Regulator SM B/3(q*)
  [qo_SM_B] -> Unit Delay omega SM A4/1
  Gain -1 Ic VSC B/1 -> [Ic_VSC_B]
  [Vdc_VSC_B] -> VSC Load B/3(Vdc)
  Gain Vb_dc VSC B/1 -> [Load_VSC_B]
  Unit Delay Vdc 12puls B/1 -> Gain 1/Vb_dc 12puls B/1
  [m_VSC_B] -> VSC B/1
  [Load_VSC_B] -> Controlled Current Source Idc VSC B/1
  Gain Ib_dc 12 puls B/1 -> Goto Idc 12puls B/1
  From Vdc 12puls B/1 -> Unit Delay Vdc 12puls B/1
  [v_hat_SM_B] -> Unit Delay omega SM A5/1
  Three-Phase Vc-Ic Measurement VSC B/2 -> Gain -1 Ic VSC B/1
  Three-Phase V0-I0 Measurement VSC B/1 -> [Vf_VSC_B]
  Vdc Measurement VSC B/1 -> [Vdc_VSC_B]
  From Idc 12puls B/1 -> Controlled Current Source 12 puls B/1
  Unit Delay Vdc VSC A/1 -> Gain 1/Vb_dc/1
  Three-Phase V0-I0 Measurement VSC B/2 -> Terminator VSC B1/1
  Gain 1/Vb_dc 12puls B/1 -> P to I 12puls B/2(v_dc)
  P to I 12puls B/1(i_dc) -> Gain Ib_dc 12 puls B/1
  Vdc Measurement 12 puls B/1 -> Goto Vdc 12 puls B/1
  Three-Phase Vc-Ic Measurement VSC B/1 -> Terminator VSC B/1
  Bus Selector7/1 -> P/Q SM B/2, [qo_SM_B]
  P to I VSC B/1(i_dc) -> Gain Vb_dc VSC B/1
  Bus Selector8/1 -> abs(v_hat) SM B/1(vd)
  "Power (3ph, Instantaneous)"/2 -> Gain5/1
  Three-Phase V-I Measurement Hotel Load A/1 -> Gain 1/Vb VMS/1, "Power (3ph, Instantaneous)"/1
  Gain2/1 -> [po_hotel_A], P/Q Hoel Load A/1
  "Power (3ph, Instantaneous)"/1 -> Gain2/1
  Gain5/1 -> P/Q Hoel Load A/2, [qo_hotel_A]
  Gain9/1 -> P/Q 12puls Load A/2, Goto qo 12puls A/1
  Three-Phase V-I Measurement 12puls  A/2 -> "Power (3ph, Instantaneous)1"/2
  Three-Phase V-I Measurement 12puls  A/1 -> "Power (3ph, Instantaneous)1"/1
  "Power (3ph, Instantaneous)1"/1 -> Gain8/1
  Gain8/1 -> Goto po 12puls A/1, P/Q 12puls Load A/1
  "Power (3ph, Instantaneous)1"/2 -> Gain9/1
  "Power (3ph, Instantaneous)2"/2 -> Gain14/1
  "Power (3ph, Instantaneous)2"/1 -> Gain13/1
  Three-Phase V-I Measurement 12puls  B/1 -> "Power (3ph, Instantaneous)2"/1
  "Power (3ph, Instantaneous)3"/2 -> Gain17/1
  Three-Phase V-I Measurement Hotel Load B/2 -> "Power (3ph, Instantaneous)3"/2
  "Power (3ph, Instantaneous)3"/1 -> Gain16/1
  Three-Phase V-I Measurement Hotel Load B/1 -> Gain 1/Vb VMS1/1, "Power (3ph, Instantaneous)3"/1
  q* VSM B/1 -> VSM A1/5(q* VSM)
  VSM A1/1(m) -> [m_VSM_B]
  [Ic_VMS_B] -> VSM A1/2(Ic)
  [Vf_VMS_B] -> VSM A1/1(Vf)
  [Vdc_VSM] -> VSM A1/3(Vdc)
  VSM A/5(v_hat_f) -> [v_hat_f_VSM_A]
  VSM A/1(m) -> [m_VSM_A]
  q* VSM A/1 -> VSM A/5(q* VSM)
  [Vf_VMS_A] -> VSM A/1(Vf)
  [Ic_VMS_A] -> VSM A/2(Ic)
  VSM A/2(omega) -> Inertia model VSM A/1, [omega_VSM_A]
  VSM A/3(p) -> Inertia model VSM A/2
  [Vdc_VSM] -> VSM A/3(Vdc)
  VSM A1/3(p) -> Inertia model VSM B/2
  VSM A1/2(omega) -> Inertia model VSM B/1, [omega_VSM_B]
  VSM A1/5(v_hat_f) -> [v_hat_f_VSM_B]
  Gain17/1 -> P/Q Hoel Load B/2, [qo_hotel_B]
  Gain16/1 -> [po_hotel_B], P/Q Hoel Load B/1
  Gain13/1 -> Goto po 12puls B/1, P/Q 12puls Load B/1
  Gain14/1 -> P/Q 12puls Load B/2, Goto qo 12puls B/1
  Automatic Voltage Regulator SM B/1(v_hat_e) -> Synchronous Machine B pu Fundamental/2, Vf SM B/1
  Diesel Generator Governor Model SM B/1(tau_dg) -> Pm SM B/1, Synchronous Machine B pu Fundamental/1
  Gain4/1 -> [po_VSM_B], P/Q VSM Load B1/1
  Three-Phase V-I Measurement VSM  B/2 -> "Power (3ph, Instantaneous)4"/2
  Gain10/1 -> [qo_VSM_B], P/Q VSM Load B1/2
  Three-Phase V-I Measurement VSM  B/1 -> "Power (3ph, Instantaneous)4"/1
  "Power (3ph, Instantaneous)4"/2 -> Gain10/1
  "Power (3ph, Instantaneous)4"/1 -> Gain4/1
  Three-Phase V-I Measurement VSM  B1/2 -> "Power (3ph, Instantaneous)5"/2
  Gain11/1 -> [po_VSM_A], P/Q VSM Load A1/1
  Three-Phase V-I Measurement VSM  B1/1 -> "Power (3ph, Instantaneous)5"/1
  "Power (3ph, Instantaneous)5"/1 -> Gain11/1
  "Power (3ph, Instantaneous)5"/2 -> Gain3/1
  Gain3/1 -> [qo_VSM_A], P/Q VSM Load A1/2
  Diesel Generator Governor Model SM A/1(tau_dg) -> Synchronous Machine A pu Fundamental/1, Pm SM A/1
  Automatic Voltage Regulator SM A/1(v_hat_e) -> Synchronous Machine A pu Fundamental/2, Vf SM A/1
  Gain19/1 -> [po_VSC_A], P/Q 12puls Load A1/1
  Three-Phase V-I Measurement VSC  A/2 -> "Power (3ph, Instantaneous)6"/2
  Gain20/1 -> [qo_VSC_A], P/Q 12puls Load A1/2
  Three-Phase V-I Measurement VSC  A/1 -> "Power (3ph, Instantaneous)6"/1
  "Power (3ph, Instantaneous)6"/2 -> Gain20/1
  "Power (3ph, Instantaneous)6"/1 -> Gain19/1
  "Power (3ph, Instantaneous)7"/1 -> Gain22/1
  Gain22/1 -> [po_VSC_B], P/Q 12puls Load A2/1
  Three-Phase V-I Measurement VSC  A1/1 -> "Power (3ph, Instantaneous)7"/1
  Gain23/1 -> [qo_VSC_B], P/Q 12puls Load A2/2
  "Power (3ph, Instantaneous)7"/2 -> Gain23/1
  Three-Phase V-I Measurement VSC  A1/2 -> "Power (3ph, Instantaneous)7"/2
  PLL grid/1(omega) -> Grid/1, [omega_grid_A]
  PLL grid/2(v_hat) -> Grid/2, [v_hat_grid_A]
  Gain 1/Vb VMS/1 -> PLL grid/1(Vo)
  Three-Phase V-I Measurement 12puls  B/2 -> "Power (3ph, Instantaneous)2"/2
  Three-Phase V-I Measurement Hotel Load A/2 -> "Power (3ph, Instantaneous)"/2
  PLL grid1/2(v_hat) -> Grid B/2, [v_hat_grid_B]
  Gain 1/Vb VMS1/1 -> PLL grid1/1(Vo)
  PLL grid1/1(omega) -> Grid B/1, [omega_grid_B]
  From27/1 -> Mux1/17
  From23/1 -> Mux1/29
  From22/1 -> Mux1/30
  From5/1 -> Mux1/1
  From6/1 -> Mux1/2
  From13/1 -> Mux1/3
  From3/1 -> Mux1/4
  From7/1 -> Mux1/5
  From8/1 -> Mux1/6
  From9/1 -> Mux1/7
  From4/1 -> Mux1/8
  From17/1 -> Mux1/9
  From11/1 -> Mux1/10
  From14/1 -> Mux1/11
  From12/1 -> Mux1/12
  From16/1 -> Mux1/13
  From15/1 -> Mux1/14
  From/1 -> Mux1/15
  From2/1 -> Mux1/16
  Mux1/1 -> To File/1
  From32/1 -> Mux1/31
  From33/1 -> Mux1/32
  From28/1 -> Mux1/18
  From20/1 -> Mux1/19
  From25/1 -> Mux1/20
  From29/1 -> Mux1/21
  From30/1 -> Mux1/22
  From31/1 -> Mux1/23
  From26/1 -> Mux1/24
  From24/1 -> Mux1/25
  From18/1 -> Mux1/26
  From21/1 -> Mux1/27
  From19/1 -> Mux1/28
  "P* SM A "/1 -> Diesel Generator Governor Model SM A/1(p*_sm)
  p* SM B/1 -> Diesel Generator Governor Model SM B/1(p*_sm)
  p* VSM A step/1 -> VSM A/4(p* VSM)
  "p* VSM B "/1 -> VSM A1/4(p* VSM)
  VSM A1/4(q) -> Terminator/1
  VSC Load B/2(p) -> Terminator2/1
  VSC Load B/3(q) -> Terminator6/1
  VSC Load A/2(p) -> Terminator9/1
  VSC Load A/3(q) -> Terminator10/1
  VSM A/4(q) -> Terminator11/1
  connections:
  Shunt resistor SM A/RConn2 -- Ground3/LConn1 -- Shunt resistor SM A/RConn1 -- Shunt resistor SM A/RConn3
  Diode 12puls A7/LConn1 -- Three-Phase Transformer (Three Windings) 12puls A/RConn5 -- Diode 12puls A10/RConn1
  Diode 12puls A3/LConn1 -- Parallel RLC Branch 12 puls A/RConn1 -- Controlled Current Source 12 puls A/LConn1 -- Vdc Measurement 12 puls A/LConn2 -- Diode 12puls A11/LConn1 -- Diode 12puls A9/LConn1 -- Diode 12puls A10/LConn1 -- Diode 12puls A5/LConn1 -- Diode 12puls A4/LConn1
  Diode 12puls A6/RConn1 -- Diode 12puls A7/RConn1 -- Controlled Current Source 12 puls A/RConn1 -- Vdc Measurement 12 puls A/LConn1 -- Parallel RLC Branch 12 puls A/LConn1 -- Diode12puls A2/RConn1 -- Diode 12puls A/RConn1 -- Diode12puls A1/RConn1 -- Diode 12puls A8/RConn1
  Diode 12puls A9/RConn1 -- Diode 12puls A6/LConn1 -- Three-Phase Transformer (Three Windings) 12puls A/RConn4
  Diode 12puls A3/RConn1 -- Three-Phase Transformer (Three Windings) 12puls A/RConn1 -- Diode 12puls A/LConn1
  Diode 12puls A8/LConn1 -- Three-Phase Transformer (Three Windings) 12puls A/RConn6 -- Diode 12puls A11/RConn1
  Diode 12puls A4/RConn1 -- Three-Phase Transformer (Three Windings) 12puls A/RConn2 -- Diode12puls A1/LConn1
  Diode12puls A2/LConn1 -- Diode 12puls A5/RConn1 -- Three-Phase Transformer (Three Windings) 12puls A/RConn3
  Three-Phase V0-I0 Measurement VSC A/RConn1 -- Filter inductor 1 VSC A/LConn1 -- Filter capacitor VSC A/LConn1
  Controlled Current Source/RConn1 -- Vdc Measurement VSC A/LConn1 -- VSC A/RConn1 -- Series RLC Branch2/LConn1
  Three-Phase V0-I0 Measurement VSC A/RConn2 -- Filter capacitor VSC A/LConn2 -- Filter inductor 1 VSC A/LConn2
  Series RLC Branch2/RConn1 -- VSC A/RConn2 -- Controlled Current Source/LConn1 -- Vdc Measurement VSC A/LConn2
  Filter capacitor VSC A/RConn2 -- Filter capacitor VSC A/RConn1 -- Filter capacitor VSC A/RConn3
  Three-Phase V0-I0 Measurement VSC A/RConn3 -- Filter capacitor VSC A/LConn3 -- Filter inductor 1 VSC A/LConn3
  Three-Phase Vc-Ic Measurement VSC A/RConn2 -- VSC A/LConn2
  Three-Phase Bus Breaker/LConn1 -- Three-Phase V-I Measurement VSC  A/LConn1 -- Three-Phase V-I Measurement VSM  B1/RConn1 -- Shunt resistor SM A/LConn1 -- Synchronous Machine A pu Fundamental/RConn1 -- Three-Phase V-I Measurement Hotel Load A/LConn1 -- Three-Phase V-I Measurement 12puls  A/LConn1
  Filter inductor 1 VSC A/RConn3 -- Three-Phase Vc-Ic Measurement VSC A/LConn3
  Filter inductor 1 VSC A/RConn2 -- Three-Phase Vc-Ic Measurement VSC A/LConn2
  Three-Phase Vc-Ic Measurement VSC A/RConn1 -- VSC A/LConn1
  Three-Phase Vc-Ic Measurement VSC A/RConn3 -- VSC A/LConn3
  Filter inductor 1 VSC A/RConn1 -- Three-Phase Vc-Ic Measurement VSC A/LConn1
  Filter inductor VSM A/LConn1 -- Three-Phase Vf Measurement VSM A/RConn1 -- Filter capacitor VSM A/LConn1
  Filter capacitor VSM A/RConn3 -- Filter capacitor VSM A/RConn1 -- Filter capacitor VSM A/RConn2
  Vdc Measurement/LConn1 -- VSC VSM B/RConn1 -- VSC VSM A/RConn1 -- DC source/RConn1
  Filter inductor VSM A/LConn3 -- Three-Phase Vf Measurement VSM A/RConn3 -- Filter capacitor VSM A/LConn3
  DC source/LConn1 -- VSC VSM B/RConn2 -- VSC VSM A/RConn2 -- Vdc Measurement/LConn2
  Filter inductor VSM A/LConn2 -- Three-Phase Vf Measurement VSM A/RConn2 -- Filter capacitor VSM A/LConn2
  Filter inductor VSM A/RConn1 -- Three-Phase Ic Measurement VSM A/LConn1
  Three-Phase Ic Measurement VSM A/RConn3 -- VSC VSM A/LConn3
  Three-Phase Ic Measurement VSM A/RConn2 -- VSC VSM A/LConn2
  Filter inductor VSM A/RConn2 -- Three-Phase Ic Measurement VSM A/LConn2
  Three-Phase Ic Measurement VSM A/RConn1 -- VSC VSM A/LConn1
  Filter inductor VSM A/RConn3 -- Three-Phase Ic Measurement VSM A/LConn3
  Three-Phase Bus Breaker/LConn3 -- Three-Phase V-I Measurement VSC  A/LConn3 -- Three-Phase V-I Measurement VSM  B1/RConn3 -- Shunt resistor SM A/LConn3 -- Synchronous Machine A pu Fundamental/RConn3 -- Three-Phase V-I Measurement Hotel Load A/LConn3 -- Three-Phase V-I Measurement 12puls  A/LConn3
  Shunt resistor SM B/LConn2 -- Synchronous Machine B pu Fundamental/RConn2 -- Three-Phase V-I Measurement Hotel Load B/LConn2 -- Three-Phase V-I Measurement 12puls  B/LConn2 -- Three-Phase V-I Measurement VSC  A1/LConn2 -- Three-Phase Bus Breaker/RConn2 -- Three-Phase V-I Measurement VSM  B/RConn2
  Three-Phase Transformer (Three Windings) 12puls B/RConn1 -- Diode 12puls B4/RConn1 -- Diode 12puls B1/LConn1
  Diode 12puls B5/LConn1 -- Diode 12puls B4/LConn1 -- Parallel RLC Branch 12 puls B/RConn1 -- Controlled Current Source 12 puls B/LConn1 -- Vdc Measurement 12 puls B/LConn2 -- Diode 12puls B12/LConn1 -- Diode 12puls B10/LConn1 -- Diode 12puls B11/LConn1 -- Diode 12puls B6/LConn1
  Filter inductor 1 VSC B/LConn3 -- Three-Phase V0-I0 Measurement VSC B/RConn3 -- Filter capacitor VSC B/LConn3
  Vdc Measurement VSC B/LConn2 -- Controlled Current Source Idc VSC B/LConn1 -- Series RLC Branch DC VSC B/RConn1 -- VSC B/RConn2
  Three-Phase Vf Measurement VSM B/RConn2 -- Filter capacitor VSM B/LConn2 -- Filter inductor VSM B/LConn2
  Filter inductor 1 VSC B/LConn2 -- Three-Phase V0-I0 Measurement VSC B/RConn2 -- Filter capacitor VSC B/LConn2
  Diode 12puls B12/RConn1 -- Diode 12puls B9/LConn1 -- Three-Phase Transformer (Three Windings) 12puls B/RConn6
  Three-Phase Transformer (Three Windings) 12puls B/RConn2 -- Diode 12puls B5/RConn1 -- Diode12puls B2/LConn1
  Three-Phase Transformer (Three Windings) 12puls B/RConn5 -- Diode 12puls B8/LConn1 -- Diode 12puls B11/RConn1
  Filter inductor VSM B/LConn1 -- Filter capacitor VSM B/LConn1 -- Three-Phase Vf Measurement VSM B/RConn1
  Shunt resistor SM B/RConn3 -- Shunt resistor SM B/RConn2 -- Shunt resistor SM B/RConn1
  Series RLC Branch DC VSC B/LConn1 -- Controlled Current Source Idc VSC B/RConn1 -- Vdc Measurement VSC B/LConn1 -- VSC B/RConn1
  Three-Phase Bus Breaker/RConn1 -- Three-Phase V-I Measurement VSM  B/RConn1 -- Three-Phase V-I Measurement VSC  A1/LConn1 -- Shunt resistor SM B/LConn1 -- Synchronous Machine B pu Fundamental/RConn1 -- Three-Phase V-I Measurement Hotel Load B/LConn1 -- Three-Phase V-I Measurement 12puls  B/LConn1
  Three-Phase V0-I0 Measurement VSC B/RConn1 -- Filter inductor 1 VSC B/LConn1 -- Filter capacitor VSC B/LConn1
  Diode12puls B3/LConn1 -- Diode 12puls B6/RConn1 -- Three-Phase Transformer (Three Windings) 12puls B/RConn3
  Diode 12puls B7/RConn1 -- Diode 12puls B8/RConn1 -- Controlled Current Source 12 puls B/RConn1 -- Vdc Measurement 12 puls B/LConn1 -- Parallel RLC Branch 12 puls B/LConn1 -- Diode12puls B3/RConn1 -- Diode 12puls B1/RConn1 -- Diode12puls B2/RConn1 -- Diode 12puls B9/RConn1
  Three-Phase Vf Measurement VSM B/RConn3 -- Filter capacitor VSM B/LConn3 -- Filter inductor VSM B/LConn3
  Diode 12puls B10/RConn1 -- Diode 12puls B7/LConn1 -- Three-Phase Transformer (Three Windings) 12puls B/RConn4
  Filter capacitor VSC B/RConn3 -- Filter capacitor VSC B/RConn2 -- Filter capacitor VSC B/RConn1
  Three-Phase Ic Measurement VSM B/RConn3 -- VSC VSM B/LConn3
  Three-Phase Vc-Ic Measurement VSC B/RConn2 -- VSC B/LConn2
  Filter inductor 1 VSC B/RConn3 -- Three-Phase Vc-Ic Measurement VSC B/LConn3
  Three-Phase Ic Measurement VSM B/RConn2 -- VSC VSM B/LConn2
  Filter inductor VSM B/RConn3 -- Three-Phase Ic Measurement VSM B/LConn3
  Filter inductor VSM B/RConn1 -- Three-Phase Ic Measurement VSM B/LConn1
  Filter inductor 1 VSC B/RConn1 -- Three-Phase Vc-Ic Measurement VSC B/LConn1
  Filter inductor VSM B/RConn2 -- Three-Phase Ic Measurement VSM B/LConn2
  Three-Phase Vc-Ic Measurement VSC B/RConn1 -- VSC B/LConn1
  Three-Phase Vc-Ic Measurement VSC B/RConn3 -- VSC B/LConn3
  Filter inductor 1 VSC B/RConn2 -- Three-Phase Vc-Ic Measurement VSC B/LConn2
  Three-Phase Ic Measurement VSM B/RConn1 -- VSC VSM B/LConn1
  Filter capacitor VSM B/RConn1 -- Filter capacitor VSM B/RConn3 -- Filter capacitor VSM B/RConn2
  Three-Phase Bus Breaker/LConn2 -- Three-Phase V-I Measurement VSC  A/LConn2 -- Three-Phase V-I Measurement VSM  B1/RConn2 -- Shunt resistor SM A/LConn2 -- Synchronous Machine A pu Fundamental/RConn2 -- Three-Phase V-I Measurement Hotel Load A/LConn2 -- Three-Phase V-I Measurement 12puls  A/LConn2
  Three-Phase Bus Breaker/RConn3 -- Three-Phase V-I Measurement VSC  A1/LConn3 -- Three-Phase V-I Measurement VSM  B/RConn3 -- Three-Phase V-I Measurement Hotel Load B/LConn3 -- Synchronous Machine B pu Fundamental/RConn3 -- Shunt resistor SM B/LConn3 -- Three-Phase V-I Measurement 12puls  B/LConn3
  Filter inductor 1 VSM A1/RConn1 -- Three-Phase Vf Measurement VSM A/LConn1
  Filter inductor 1 VSM A1/RConn2 -- Three-Phase Vf Measurement VSM A/LConn2
  Filter inductor 1 VSM A1/RConn3 -- Three-Phase Vf Measurement VSM A/LConn3
  Filter inductor 1 VSC A1/RConn1 -- Three-Phase V0-I0 Measurement VSC A/LConn1
  Filter inductor 1 VSC A1/RConn2 -- Three-Phase V0-I0 Measurement VSC A/LConn2
  Filter inductor 1 VSC A1/RConn3 -- Three-Phase V0-I0 Measurement VSC A/LConn3
  Filter inductor 1 VSM B1/RConn1 -- Three-Phase Vf Measurement VSM B/LConn1
  Filter inductor 1 VSM B1/RConn2 -- Three-Phase Vf Measurement VSM B/LConn2
  Filter inductor 1 VSM B1/RConn3 -- Three-Phase Vf Measurement VSM B/LConn3
  Filter inductor 1 VSC B1/RConn3 -- Three-Phase V0-I0 Measurement VSC B/LConn3
  Filter inductor 1 VSC B1/RConn2 -- Three-Phase V0-I0 Measurement VSC B/LConn2
  Filter inductor 1 VSC B1/RConn1 -- Three-Phase V0-I0 Measurement VSC B/LConn1
  Three-Phase Parallel RLC Load Hotel Load A/LConn2 -- Three-Phase V-I Measurement Hotel Load A/RConn2
  Three-Phase Parallel RLC Load Hotel Load A/LConn1 -- Three-Phase V-I Measurement Hotel Load A/RConn1
  Three-Phase Parallel RLC Load Hotel Load A/LConn3 -- Three-Phase V-I Measurement Hotel Load A/RConn3
  Three-Phase V-I Measurement 12puls  A/RConn2 -- Three-Phase Transformer (Three Windings) 12puls A/LConn2
  Three-Phase V-I Measurement 12puls  A/RConn3 -- Three-Phase Transformer (Three Windings) 12puls A/LConn3
  Three-Phase V-I Measurement 12puls  A/RConn1 -- Three-Phase Transformer (Three Windings) 12puls A/LConn1
  Three-Phase V-I Measurement 12puls  B/RConn2 -- Three-Phase Transformer (Three Windings) 12puls B/LConn2
  Three-Phase V-I Measurement 12puls  B/RConn3 -- Three-Phase Transformer (Three Windings) 12puls B/LConn3
  Three-Phase Transformer (Three Windings) 12puls B/LConn1 -- Three-Phase V-I Measurement 12puls  B/RConn1
  Three-Phase Parallel RLC Load Hotel Load B/LConn3 -- Three-Phase V-I Measurement Hotel Load B/RConn3
  Three-Phase Parallel RLC Load Hotel Load B/LConn2 -- Three-Phase V-I Measurement Hotel Load B/RConn2
  Three-Phase Parallel RLC Load Hotel Load B/LConn1 -- Three-Phase V-I Measurement Hotel Load B/RConn1
  Three-Phase V-I Measurement VSM  B/LConn1 -- Filter inductor 1 VSM B1/LConn1
  Three-Phase V-I Measurement VSM  B/LConn2 -- Filter inductor 1 VSM B1/LConn2
  Three-Phase V-I Measurement VSM  B/LConn3 -- Filter inductor 1 VSM B1/LConn3
  Filter inductor 1 VSM A1/LConn3 -- Three-Phase V-I Measurement VSM  B1/LConn3
  Filter inductor 1 VSM A1/LConn1 -- Three-Phase V-I Measurement VSM  B1/LConn1
  Filter inductor 1 VSM A1/LConn2 -- Three-Phase V-I Measurement VSM  B1/LConn2
  Three-Phase V-I Measurement VSC  A/RConn3 -- Filter inductor 1 VSC A1/LConn3
  Three-Phase V-I Measurement VSC  A/RConn2 -- Filter inductor 1 VSC A1/LConn2
  Three-Phase V-I Measurement VSC  A/RConn1 -- Filter inductor 1 VSC A1/LConn1
  Three-Phase V-I Measurement VSC  A1/RConn1 -- Filter inductor 1 VSC B1/LConn1
  Three-Phase V-I Measurement VSC  A1/RConn3 -- Filter inductor 1 VSC B1/LConn3
  Three-Phase V-I Measurement VSC  A1/RConn2 -- Filter inductor 1 VSC B1/LConn2
